simulink library "snn_champions_lib"  (R2026a)
settings: Solver=VariableStepAuto
(part 1 of 24)
settings Model: Creator=user poco smart  LastModifiedBy=user poco smart

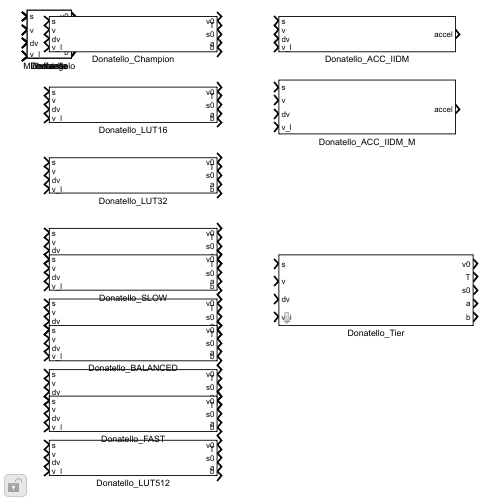
[thumbnail: Simulink's stored preview of the top-level diagram]
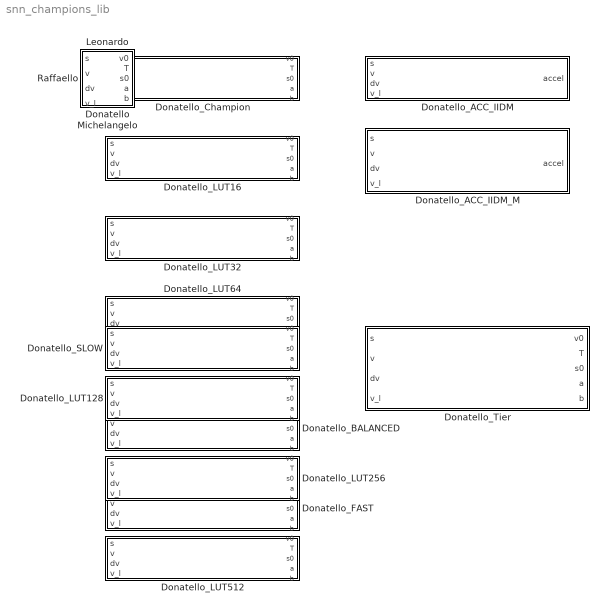
== system snn_champions_lib ==
  Donatello : Subsystem
  Donatello_ACC_IIDM : Subsystem  Description=|
      | Donatello_ACC_IIDM - campione Donatello (LUT-64) + modello ACC-IIDM open-loop.
      | 
      | HDL-READY dal 2026-07-16 (SP3): HDL Coder genera il VHDL dal solo .slx, con DualPortRAM (cioe'
      |    l'architettura time-mux del deployato). Fino a quella data l'IIDM girava in double e HDL
      |    Coder rifiutava il blocco con 14 errori; ora l'IIDM e' fixed-point (acc_types, Q10.8).
      |    Non servirono LUT: sqrt/tanh/x^4 sono NATIVI in HDL Coder e la divisione passa con
      |    RoundingMethod 'Zero'. Cancello: run_block_hdl_gate.
      | 
      | ⚠️ HDL-READY NON VUOL DIRE DEPLOYATO: il bitstream PYNQ-Z1 resta la sola SNN. Questo blocco da'
      |    il costo in silicio del controllore COMPLETO (rete + legge di controllo), che e' cio' che si
      |    confronta con un MPC. Dettagli: document/SP3_ACC_IIDM_HDL.md.
      | 
      | FUNZIONE
      |   Catena completa stato -> azione: la SNN stima i 5 parametri IDM, il modello ACC-IIDM li usa
      |   per calcolare l'accelerazione. Serve a testare la rete dentro un modello di car-following.
      | 
      | INGRESSI (fisici, fixed con >=20 bit frazionari - interporre un Data Type Conversion)
      |   s [m] · v [m/s] · dv [m/s] (= v - v_l) · v_l [m/s]
      | USCITA
      |   accel [m/s^2]
      | 
      | LOOP APERTO
      |   Il blocco NON integra v ne' s: li riceve. Il loop lo chiude il sistema che testa (la velocita'
      |   effettiva puo' essere alterata a valle). L'unico stato interno e' il filtro OU che stima a_l.
      | 
      | SEMANTICA E RATE
      |   1 cambio d'ingresso = 1 control-step = DT 0.1 s. Ogni ingresso va tenuto per almeno ~341
      |   campioni (la SNN e' time-multiplexata: 1 neurone/clock). L'IIDM gira una volta per
      |   control-step, quando i parametri si rinfrescano.
      | 
      | RIFERIMENTI
      |   docs/superpowers/specs/2026-07-14-sp2-donatello-acc-iidm-design.md · document/SP2_ACC_IIDM.md
      |   Rigenerazione: build_hdl_variants.m (NON modificare la chart a mano)
  Donatello_ACC_IIDM_M : Subsystem  Description=|
      | Donatello_ACC_IIDM_M - Donatello (LUT-64) + ACC-IIDM con le 5 divisioni SEQUENZIATE.
      | 
      | COS'E' (SP4-M-FSM #2a)
      |   Variante di Donatello_ACC_IIDM: le 5 divisioni a divisore variabile dell'IIDM non sono piu' 5
      |   divisori combinatori INCATENATI (1077 livelli logici, Fmax 2,0 MHz), ma UNA sola divide()
      |   riusata da una macchina a stati -- una divisione per ciclo. Scopo: TAGLIARE L'AREA tenendo
      |   dmax=0. Il path critico resta una divisione combinatoria: questo blocco NON punta agli 11,65 MHz
      |   (per quelli servirebbe un divisore sequenziale, studio #2b: SP4_ACC_IIDM_FAST.md).
      | 
      | BIT-IDENTICO A Donatello_ACC_IIDM (SP3)
      |   La matematica e' la stessa, solo distribuita nel tempo: nessuna approssimazione. Garantito da
      |   tre cancelli sul dataset intero:
      |     G1  il blocco Divide (ShiftAdd, RndMeth Zero, Q10.8) e' bit-identico a divide() di SP3
      |         -> dmax=0 su 300.000 coppie (num,den) reali; sensibile (RndMeth Nearest -> 1 LSB).
      |     G2  le funzioni-fase (iidm_prep/nd/use/final) == acc_iidm_open -> dmax=0 su 60.000/60.000
      |         control-step; sensibile (q2 al posto di q3 -> 1990/2000 divergenti).
      |     G3  questo blocco == il model acc_iidm_fsm (run_block_acciidm_m_test).
      | 
      | INGRESSI (fisici, fixed con >=20 bit frazionari - interporre un Data Type Conversion)
      |   s [m] · v [m/s] · dv [m/s] (= v - v_l) · v_l [m/s]
      | USCITA
      |   accel [m/s^2]
      | 
      | ⚠️ VINCOLO DI RATE (DIVERSO da Donatello_ACC_IIDM)
      |   Una inferenza costa la SNN time-mux (~341 clock) PIU' 5 cicli, uno per divisione. Ogni ingresso
      |   va quindi tenuto per PIU' campioni che nel blocco SP3 (~341): il valore esatto lo MISURA
      |   run_block_acciidm_m_test (non e' assunto). Sull'FPGA e' irrilevante: un control-step da 0,1 s
      |   dura 800.000 clock a 8 MHz.
      | 
      | SEMANTICA
      |   1 cambio d'ingresso = 1 inferenza (edge-triggered, niente start/done esposti: uno start
      |   scollegato sarebbe un fallimento SILENZIOSO -- HDL_PHASE §3.1.2). Le uscite mantengono l'ultimo
      |   valore fino all'inferenza successiva.
      | 
      | RIFERIMENTI
      |   docs/superpowers/specs/2026-07-16-acc-iidm-fsm-design.md · document/SP4_ACC_IIDM_FAST.md
      |   Rigenerazione: build_hdl_variants.m (NON modificare la chart a mano)
  Donatello_BALANCED : Subsystem  Description=|
      | Donatello_BALANCED - SNN car-following (champion Donatello), architettura SPLITPIPE (SNN+decode come due
      | entita' di sintesi, con registro sugli operandi del normalize). Tier dello Studio Trade-off (Blocco A).
      | 
      | CONFIGURAZIONE: R5 (SNN 5 stadi) + decode p3  -> tier COMPROMESSO (~58 MHz io-timed)
      | Decode della sigmoide via LUT a 64 punti. I tre tier danno gli STESSI 5 parametri (bit-exact fra loro),
      | differiscono per latenza (342/364/406 clock) e profilo di risorse/Fmax.
      | 
      | INGRESSI (fisici, fixed >=20 bit frazionari): s [m], v [m/s], dv [m/s] (sat +-20), v_l [m/s].
      | USCITE (parametri IDM): v0, T, s0, a, b.  1 campione = 1 inferenza (edge-triggered), niente start/done.
      | 
      | SELF-CONTAINED: nessun .m esterno; HDL Coder genera il VHDL dal solo blocco (time-mux, DualPortRAM).
      | VERIFICHE: run_block_hdl_gate (self-contained) · run_block_traj_test (dmax=0).
      | Rigenerazione: build_tier_blocks.m (NON modificare la chart a mano).
  Donatello_Champion : Subsystem  Description=|
      | Donatello_Champion - SNN car-following (champion Donatello), architettura B2 time-multiplexata.
      | 
      | FUNZIONE
      |   Stima i 5 parametri IDM del veicolo osservato a partire dallo stato di car-following.
      | 
      | INGRESSI (grandezze fisiche)
      |   s    [m]    spaziatura dal veicolo che precede
      |   v    [m/s]  velocita' del veicolo
      |   dv   [m/s]  velocita' relativa (v - v_l); saturata internamente a +-20
      |   v_l  [m/s]  velocita' del veicolo che precede
      | 
      | USCITE (parametri IDM stimati)
      |   v0 [m/s]  ·  T [s]  ·  s0 [m]  ·  a [m/s^2]  ·  b [m/s^2]
      | 
      | TIPI DI DATO (vincolo)
      |   Gli ingressi devono essere fixed-point con ALMENO 20 bit frazionari, ad esempio
      |   fixdt(1,32,20). Il tipo double NON e' ammesso: non e' sintetizzabile e il blocco non
      |   compila. Per sorgenti in double (es. le traiettorie di test_dataset.mat) interporre un
      |   blocco "Data Type Conversion". Con meno di 20 bit frazionari il blocco funziona ma non
      |   e' bit-exact rispetto al riferimento software (la normalizzazione devia di 1 LSB circa
      |   1 volta ogni 25 campioni, il che fa cambiare uno spike).
      | 
      | SEMANTICA: 1 campione = 1 inferenza
      |   Una inferenza viene avviata a ogni cambio degli ingressi (edge-triggered). Il blocco non
      |   espone start/done. Le uscite mantengono l'ultimo valore calcolato fino all'inferenza
      |   successiva.
      | 
      | VINCOLO DI RATE
      |   L'architettura time-multiplexata elabora un neurone per clock: una inferenza richiede
      |   circa 341 campioni. Ogni ingresso va quindi mantenuto per almeno 341 passi di simulazione.
      |   Il valore esatto e' irrilevante: qualunque durata >= 341 e' corretta. Sull'FPGA il vincolo
      |   e' soddisfatto con ampio margine (un control-step da 0.1 s dura 800.000 clock e l'inferenza
      |   ne usa 341, pari allo 0,04%).
      | 
      | LIMITE NOTO
      |   Se due campioni consecutivi hanno tutti e quattro gli ingressi bit-identici, il cambio non
      |   viene rilevato e una inferenza viene saltata.
      | 
      | IMPLEMENTAZIONE
      |   IL CAMPIONE: e' esattamente cio' che va sull'FPGA (stesso decode del top deployato snn_top_b2). Decode della sigmoide via LUT a 64 punti. Perche' 64: lo studio DECODE_LUT_SWEEP.md ha misurato che l'accuratezza e' piatta (~84%) su N=16..512, e che 64 e' la LUT piu' piccola il cui errore d'approssimazione su v0 (0.0114) resta SOTTO l'errore di quantizzazione fixed gia' accettato (0.028) -> il decode non diventa la fonte d'errore dominante. Rispetto ai 256 punti usati fino al 2026-07-14: accuratezza identica (83.98 vs 83.97) e -288 LUT sul top (4630 -> 4342). Nota: funzionalmente IDENTICO al blocco Donatello_LUT64 (qui il nome dice cosa si deploya, li' che e' una variante di studio).
      |   Il forward e' il B2 time-multiplexato, identico all'architettura del bitstream PYNQ-Z1.
      |   Il blocco e' SELF-CONTAINED: non richiede alcun file .m esterno. HDL Coder genera il VHDL
      |   direttamente dal blocco (architettura time-mux, con DualPortRAM).
      | 
      | VERIFICHE
      |   run_block_hdl_gate   - copia il solo .slx in una cartella isolata, rimuove matlab/ dal path
      |                          e lancia makehdl: dimostra che il VHDL si genera su un altro PC.
      |   run_block_traj_test  - pilota il blocco con le traiettorie di test_dataset.mat e verifica
      |                          che i parametri coincidano con il riferimento (dmax = 0).
      | 
      | RIFERIMENTI
      |   document/HDL_PHASE.md         §3.1 contratto d'interfaccia, §3.1.4 edge-trigger e rate
      |   document/DECODE_LUT_SWEEP.md  §6 blocchi e verifiche
      |   Rigenerazione: build_hdl_variants.m (NON modificare la chart a mano)
  Donatello_FAST : Subsystem  Description=|
      | Donatello_FAST - SNN car-following (champion Donatello), architettura SPLITPIPE (SNN+decode come due
      | entita' di sintesi, con registro sugli operandi del normalize). Tier dello Studio Trade-off (Blocco A).
      | 
      | CONFIGURAZIONE: R9 (SNN 9 stadi) + decode p5      -> tier MARGINE MASSIMO (~74 MHz io-timed)
      | Decode della sigmoide via LUT a 64 punti. I tre tier danno gli STESSI 5 parametri (bit-exact fra loro),
      | differiscono per latenza (342/364/406 clock) e profilo di risorse/Fmax.
      | 
      | INGRESSI (fisici, fixed >=20 bit frazionari): s [m], v [m/s], dv [m/s] (sat +-20), v_l [m/s].
      | USCITE (parametri IDM): v0, T, s0, a, b.  1 campione = 1 inferenza (edge-triggered), niente start/done.
      | 
      | SELF-CONTAINED: nessun .m esterno; HDL Coder genera il VHDL dal solo blocco (time-mux, DualPortRAM).
      | VERIFICHE: run_block_hdl_gate (self-contained) · run_block_traj_test (dmax=0).
      | Rigenerazione: build_tier_blocks.m (NON modificare la chart a mano).
  Donatello_LUT128 : Subsystem  Description=|
      | Donatello_LUT128 - SNN car-following (champion Donatello), architettura B2 time-multiplexata.
      | 
      | FUNZIONE
      |   Stima i 5 parametri IDM del veicolo osservato a partire dallo stato di car-following.
      | 
      | INGRESSI (grandezze fisiche)
      |   s    [m]    spaziatura dal veicolo che precede
      |   v    [m/s]  velocita' del veicolo
      |   dv   [m/s]  velocita' relativa (v - v_l); saturata internamente a +-20
      |   v_l  [m/s]  velocita' del veicolo che precede
      | 
      | USCITE (parametri IDM stimati)
      |   v0 [m/s]  ·  T [s]  ·  s0 [m]  ·  a [m/s^2]  ·  b [m/s^2]
      | 
      | TIPI DI DATO (vincolo)
      |   Gli ingressi devono essere fixed-point con ALMENO 20 bit frazionari, ad esempio
      |   fixdt(1,32,20). Il tipo double NON e' ammesso: non e' sintetizzabile e il blocco non
      |   compila. Per sorgenti in double (es. le traiettorie di test_dataset.mat) interporre un
      |   blocco "Data Type Conversion". Con meno di 20 bit frazionari il blocco funziona ma non
      |   e' bit-exact rispetto al riferimento software (la normalizzazione devia di 1 LSB circa
      |   1 volta ogni 25 campioni, il che fa cambiare uno spike).
      | 
      | SEMANTICA: 1 campione = 1 inferenza
      |   Una inferenza viene avviata a ogni cambio degli ingressi (edge-triggered). Il blocco non
      |   espone start/done. Le uscite mantengono l'ultimo valore calcolato fino all'inferenza
      |   successiva.
      | 
      | VINCOLO DI RATE
      |   L'architettura time-multiplexata elabora un neurone per clock: una inferenza richiede
      |   circa 341 campioni. Ogni ingresso va quindi mantenuto per almeno 341 passi di simulazione.
      |   Il valore esatto e' irrilevante: qualunque durata >= 341 e' corretta. Sull'FPGA il vincolo
      |   e' soddisfatto con ampio margine (un control-step da 0.1 s dura 800.000 clock e l'inferenza
      |   ne usa 341, pari allo 0,04%).
      | 
      | LIMITE NOTO
      |   Se due campioni consecutivi hanno tutti e quattro gli ingressi bit-identici, il cambio non
      |   viene rilevato e una inferenza viene saltata.
      | 
      | IMPLEMENTAZIONE
      |   Decode della sigmoide via LUT a 128 punti (snn_decode_lut). Variante per lo studio del compromesso dimensione-LUT / accuratezza / risorse: l'accuratezza e' piatta (~84%) su N=16..512 mentre le LUT di sintesi crescono da 520 a 1732 (vedi document/DECODE_LUT_SWEEP.md). Il forward e' identico in tutte le varianti.
      |   Il forward e' il B2 time-multiplexato, identico all'architettura del bitstream PYNQ-Z1.
      |   Il blocco e' SELF-CONTAINED: non richiede alcun file .m esterno. HDL Coder genera il VHDL
      |   direttamente dal blocco (architettura time-mux, con DualPortRAM).
      | 
      | VERIFICHE
      |   run_block_hdl_gate   - copia il solo .slx in una cartella isolata, rimuove matlab/ dal path
      |                          e lancia makehdl: dimostra che il VHDL si genera su un altro PC.
      |   run_block_traj_test  - pilota il blocco con le traiettorie di test_dataset.mat e verifica
      |                          che i parametri coincidano con il riferimento (dmax = 0).
      | 
      | RIFERIMENTI
      |   document/HDL_PHASE.md         §3.1 contratto d'interfaccia, §3.1.4 edge-trigger e rate
      |   document/DECODE_LUT_SWEEP.md  §6 blocchi e verifiche
      |   Rigenerazione: build_hdl_variants.m (NON modificare la chart a mano)
  Donatello_LUT16 : Subsystem  Description=|
      | Donatello_LUT16 - SNN car-following (champion Donatello), architettura B2 time-multiplexata.
      | 
      | FUNZIONE
      |   Stima i 5 parametri IDM del veicolo osservato a partire dallo stato di car-following.
      | 
      | INGRESSI (grandezze fisiche)
      |   s    [m]    spaziatura dal veicolo che precede
      |   v    [m/s]  velocita' del veicolo
      |   dv   [m/s]  velocita' relativa (v - v_l); saturata internamente a +-20
      |   v_l  [m/s]  velocita' del veicolo che precede
      | 
      | USCITE (parametri IDM stimati)
      |   v0 [m/s]  ·  T [s]  ·  s0 [m]  ·  a [m/s^2]  ·  b [m/s^2]
      | 
      | TIPI DI DATO (vincolo)
      |   Gli ingressi devono essere fixed-point con ALMENO 20 bit frazionari, ad esempio
      |   fixdt(1,32,20). Il tipo double NON e' ammesso: non e' sintetizzabile e il blocco non
      |   compila. Per sorgenti in double (es. le traiettorie di test_dataset.mat) interporre un
      |   blocco "Data Type Conversion". Con meno di 20 bit frazionari il blocco funziona ma non
      |   e' bit-exact rispetto al riferimento software (la normalizzazione devia di 1 LSB circa
      |   1 volta ogni 25 campioni, il che fa cambiare uno spike).
      | 
      | SEMANTICA: 1 campione = 1 inferenza
      |   Una inferenza viene avviata a ogni cambio degli ingressi (edge-triggered). Il blocco non
      |   espone start/done. Le uscite mantengono l'ultimo valore calcolato fino all'inferenza
      |   successiva.
      | 
      | VINCOLO DI RATE
      |   L'architettura time-multiplexata elabora un neurone per clock: una inferenza richiede
      |   circa 341 campioni. Ogni ingresso va quindi mantenuto per almeno 341 passi di simulazione.
      |   Il valore esatto e' irrilevante: qualunque durata >= 341 e' corretta. Sull'FPGA il vincolo
      |   e' soddisfatto con ampio margine (un control-step da 0.1 s dura 800.000 clock e l'inferenza
      |   ne usa 341, pari allo 0,04%).
      | 
      | LIMITE NOTO
      |   Se due campioni consecutivi hanno tutti e quattro gli ingressi bit-identici, il cambio non
      |   viene rilevato e una inferenza viene saltata.
      | 
      | IMPLEMENTAZIONE
      |   Decode della sigmoide via LUT a 16 punti (snn_decode_lut). Variante per lo studio del compromesso dimensione-LUT / accuratezza / risorse: l'accuratezza e' piatta (~84%) su N=16..512 mentre le LUT di sintesi crescono da 520 a 1732 (vedi document/DECODE_LUT_SWEEP.md). Il forward e' identico in tutte le varianti.
      |   Il forward e' il B2 time-multiplexato, identico all'architettura del bitstream PYNQ-Z1.
      |   Il blocco e' SELF-CONTAINED: non richiede alcun file .m esterno. HDL Coder genera il VHDL
      |   direttamente dal blocco (architettura time-mux, con DualPortRAM).
      | 
      | VERIFICHE
      |   run_block_hdl_gate   - copia il solo .slx in una cartella isolata, rimuove matlab/ dal path
      |                          e lancia makehdl: dimostra che il VHDL si genera su un altro PC.
      |   run_block_traj_test  - pilota il blocco con le traiettorie di test_dataset.mat e verifica
      |                          che i parametri coincidano con il riferimento (dmax = 0).
      | 
      | RIFERIMENTI
      |   document/HDL_PHASE.md         §3.1 contratto d'interfaccia, §3.1.4 edge-trigger e rate
      |   document/DECODE_LUT_SWEEP.md  §6 blocchi e verifiche
      |   Rigenerazione: build_hdl_variants.m (NON modificare la chart a mano)
  Donatello_LUT256 : Subsystem  Description=|
      | Donatello_LUT256 - SNN car-following (champion Donatello), architettura B2 time-multiplexata.
      | 
      | FUNZIONE
      |   Stima i 5 parametri IDM del veicolo osservato a partire dallo stato di car-following.
      | 
      | INGRESSI (grandezze fisiche)
      |   s    [m]    spaziatura dal veicolo che precede
      |   v    [m/s]  velocita' del veicolo
      |   dv   [m/s]  velocita' relativa (v - v_l); saturata internamente a +-20
      |   v_l  [m/s]  velocita' del veicolo che precede
      | 
      | USCITE (parametri IDM stimati)
      |   v0 [m/s]  ·  T [s]  ·  s0 [m]  ·  a [m/s^2]  ·  b [m/s^2]
      | 
      | TIPI DI DATO (vincolo)
      |   Gli ingressi devono essere fixed-point con ALMENO 20 bit frazionari, ad esempio
      |   fixdt(1,32,20). Il tipo double NON e' ammesso: non e' sintetizzabile e il blocco non
      |   compila. Per sorgenti in double (es. le traiettorie di test_dataset.mat) interporre un
      |   blocco "Data Type Conversion". Con meno di 20 bit frazionari il blocco funziona ma non
      |   e' bit-exact rispetto al riferimento software (la normalizzazione devia di 1 LSB circa
      |   1 volta ogni 25 campioni, il che fa cambiare uno spike).
      | 
      | SEMANTICA: 1 campione = 1 inferenza
      |   Una inferenza viene avviata a ogni cambio degli ingressi (edge-triggered). Il blocco non
      |   espone start/done. Le uscite mantengono l'ultimo valore calcolato fino all'inferenza
      |   successiva.
      | 
      | VINCOLO DI RATE
      |   L'architettura time-multiplexata elabora un neurone per clock: una inferenza richiede
      |   circa 341 campioni. Ogni ingresso va quindi mantenuto per almeno 341 passi di simulazione.
      |   Il valore esatto e' irrilevante: qualunque durata >= 341 e' corretta. Sull'FPGA il vincolo
      |   e' soddisfatto con ampio margine (un control-step da 0.1 s dura 800.000 clock e l'inferenza
      |   ne usa 341, pari allo 0,04%).
      | 
      | LIMITE NOTO
      |   Se due campioni consecutivi hanno tutti e quattro gli ingressi bit-identici, il cambio non
      |   viene rilevato e una inferenza viene saltata.
      | 
      | IMPLEMENTAZIONE
      |   Decode della sigmoide via LUT a 256 punti (snn_decode_lut). Variante per lo studio del compromesso dimensione-LUT / accuratezza / risorse: l'accuratezza e' piatta (~84%) su N=16..512 mentre le LUT di sintesi crescono da 520 a 1732 (vedi document/DECODE_LUT_SWEEP.md). Il forward e' identico in tutte le varianti.
      |   Il forward e' il B2 time-multiplexato, identico all'architettura del bitstream PYNQ-Z1.
      |   Il blocco e' SELF-CONTAINED: non richiede alcun file .m esterno. HDL Coder genera il VHDL
      |   direttamente dal blocco (architettura time-mux, con DualPortRAM).
      | 
      | VERIFICHE
      |   run_block_hdl_gate   - copia il solo .slx in una cartella isolata, rimuove matlab/ dal path
      |                          e lancia makehdl: dimostra che il VHDL si genera su un altro PC.
      |   run_block_traj_test  - pilota il blocco con le traiettorie di test_dataset.mat e verifica
      |                          che i parametri coincidano con il riferimento (dmax = 0).
      | 
      | RIFERIMENTI
      |   document/HDL_PHASE.md         §3.1 contratto d'interfaccia, §3.1.4 edge-trigger e rate
      |   document/DECODE_LUT_SWEEP.md  §6 blocchi e verifiche
      |   Rigenerazione: build_hdl_variants.m (NON modificare la chart a mano)
  Donatello_LUT32 : Subsystem  Description=|
      | Donatello_LUT32 - SNN car-following (champion Donatello), architettura B2 time-multiplexata.
      | 
      | FUNZIONE
      |   Stima i 5 parametri IDM del veicolo osservato a partire dallo stato di car-following.
      | 
      | INGRESSI (grandezze fisiche)
      |   s    [m]    spaziatura dal veicolo che precede
      |   v    [m/s]  velocita' del veicolo
      |   dv   [m/s]  velocita' relativa (v - v_l); saturata internamente a +-20
      |   v_l  [m/s]  velocita' del veicolo che precede
      | 
      | USCITE (parametri IDM stimati)
      |   v0 [m/s]  ·  T [s]  ·  s0 [m]  ·  a [m/s^2]  ·  b [m/s^2]
      | 
      | TIPI DI DATO (vincolo)
      |   Gli ingressi devono essere fixed-point con ALMENO 20 bit frazionari, ad esempio
      |   fixdt(1,32,20). Il tipo double NON e' ammesso: non e' sintetizzabile e il blocco non
      |   compila. Per sorgenti in double (es. le traiettorie di test_dataset.mat) interporre un
      |   blocco "Data Type Conversion". Con meno di 20 bit frazionari il blocco funziona ma non
      |   e' bit-exact rispetto al riferimento software (la normalizzazione devia di 1 LSB circa
      |   1 volta ogni 25 campioni, il che fa cambiare uno spike).
      | 
      | SEMANTICA: 1 campione = 1 inferenza
      |   Una inferenza viene avviata a ogni cambio degli ingressi (edge-triggered). Il blocco non
      |   espone start/done. Le uscite mantengono l'ultimo valore calcolato fino all'inferenza
      |   successiva.
      | 
      | VINCOLO DI RATE
      |   L'architettura time-multiplexata elabora un neurone per clock: una inferenza richiede
      |   circa 341 campioni. Ogni ingresso va quindi mantenuto per almeno 341 passi di simulazione.
      |   Il valore esatto e' irrilevante: qualunque durata >= 341 e' corretta. Sull'FPGA il vincolo
      |   e' soddisfatto con ampio margine (un control-step da 0.1 s dura 800.000 clock e l'inferenza
      |   ne usa 341, pari allo 0,04%).
      | 
      | LIMITE NOTO
      |   Se due campioni consecutivi hanno tutti e quattro gli ingressi bit-identici, il cambio non
      |   viene rilevato e una inferenza viene saltata.
      | 
      | IMPLEMENTAZIONE
      |   Decode della sigmoide via LUT a 32 punti (snn_decode_lut). Variante per lo studio del compromesso dimensione-LUT / accuratezza / risorse: l'accuratezza e' piatta (~84%) su N=16..512 mentre le LUT di sintesi crescono da 520 a 1732 (vedi document/DECODE_LUT_SWEEP.md). Il forward e' identico in tutte le varianti.
      |   Il forward e' il B2 time-multiplexato, identico all'architettura del bitstream PYNQ-Z1.
      |   Il blocco e' SELF-CONTAINED: non richiede alcun file .m esterno. HDL Coder genera il VHDL
      |   direttamente dal blocco (architettura time-mux, con DualPortRAM).
      | 
      | VERIFICHE
      |   run_block_hdl_gate   - copia il solo .slx in una cartella isolata, rimuove matlab/ dal path
      |                          e lancia makehdl: dimostra che il VHDL si genera su un altro PC.
      |   run_block_traj_test  - pilota il blocco con le traiettorie di test_dataset.mat e verifica
      |                          che i parametri coincidano con il riferimento (dmax = 0).
      | 
      | RIFERIMENTI
      |   document/HDL_PHASE.md         §3.1 contratto d'interfaccia, §3.1.4 edge-trigger e rate
      |   document/DECODE_LUT_SWEEP.md  §6 blocchi e verifiche
      |   Rigenerazione: build_hdl_variants.m (NON modificare la chart a mano)
  Donatello_LUT512 : Subsystem  Description=|
      | Donatello_LUT512 - SNN car-following (champion Donatello), architettura B2 time-multiplexata.
      | 
      | FUNZIONE
      |   Stima i 5 parametri IDM del veicolo osservato a partire dallo stato di car-following.
      | 
      | INGRESSI (grandezze fisiche)
      |   s    [m]    spaziatura dal veicolo che precede
      |   v    [m/s]  velocita' del veicolo
      |   dv   [m/s]  velocita' relativa (v - v_l); saturata internamente a +-20
      |   v_l  [m/s]  velocita' del veicolo che precede
      | 
      | USCITE (parametri IDM stimati)
      |   v0 [m/s]  ·  T [s]  ·  s0 [m]  ·  a [m/s^2]  ·  b [m/s^2]
      | 
      | TIPI DI DATO (vincolo)
      |   Gli ingressi devono essere fixed-point con ALMENO 20 bit frazionari, ad esempio
      |   fixdt(1,32,20). Il tipo double NON e' ammesso: non e' sintetizzabile e il blocco non
      |   compila. Per sorgenti in double (es. le traiettorie di test_dataset.mat) interporre un
      |   blocco "Data Type Conversion". Con meno di 20 bit frazionari il blocco funziona ma non
      |   e' bit-exact rispetto al riferimento software (la normalizzazione devia di 1 LSB circa
      |   1 volta ogni 25 campioni, il che fa cambiare uno spike).
      | 
      | SEMANTICA: 1 campione = 1 inferenza
      |   Una inferenza viene avviata a ogni cambio degli ingressi (edge-triggered). Il blocco non
      |   espone start/done. Le uscite mantengono l'ultimo valore calcolato fino all'inferenza
      |   successiva.
      | 
      | VINCOLO DI RATE
      |   L'architettura time-multiplexata elabora un neurone per clock: una inferenza richiede
      |   circa 341 campioni. Ogni ingresso va quindi mantenuto per almeno 341 passi di simulazione.
      |   Il valore esatto e' irrilevante: qualunque durata >= 341 e' corretta. Sull'FPGA il vincolo
      |   e' soddisfatto con ampio margine (un control-step da 0.1 s dura 800.000 clock e l'inferenza
      |   ne usa 341, pari allo 0,04%).
      | 
      | LIMITE NOTO
      |   Se due campioni consecutivi hanno tutti e quattro gli ingressi bit-identici, il cambio non
      |   viene rilevato e una inferenza viene saltata.
      | 
      | IMPLEMENTAZIONE
      |   Decode della sigmoide via LUT a 512 punti (snn_decode_lut). Variante per lo studio del compromesso dimensione-LUT / accuratezza / risorse: l'accuratezza e' piatta (~84%) su N=16..512 mentre le LUT di sintesi crescono da 520 a 1732 (vedi document/DECODE_LUT_SWEEP.md). Il forward e' identico in tutte le varianti.
      |   Il forward e' il B2 time-multiplexato, identico all'architettura del bitstream PYNQ-Z1.
      |   Il blocco e' SELF-CONTAINED: non richiede alcun file .m esterno. HDL Coder genera il VHDL
      |   direttamente dal blocco (architettura time-mux, con DualPortRAM).
      | 
      | VERIFICHE
      |   run_block_hdl_gate   - copia il solo .slx in una cartella isolata, rimuove matlab/ dal path
      |                          e lancia makehdl: dimostra che il VHDL si genera su un altro PC.
      |   run_block_traj_test  - pilota il blocco con le traiettorie di test_dataset.mat e verifica
      |                          che i parametri coincidano con il riferimento (dmax = 0).
      | 
      | RIFERIMENTI
      |   document/HDL_PHASE.md         §3.1 contratto d'interfaccia, §3.1.4 edge-trigger e rate
      |   document/DECODE_LUT_SWEEP.md  §6 blocchi e verifiche
      |   Rigenerazione: build_hdl_variants.m (NON modificare la chart a mano)
  Donatello_LUT64 : Subsystem  Description=|
      | Donatello_LUT64 - SNN car-following (champion Donatello), architettura B2 time-multiplexata.
      | 
      | FUNZIONE
      |   Stima i 5 parametri IDM del veicolo osservato a partire dallo stato di car-following.
      | 
      | INGRESSI (grandezze fisiche)
      |   s    [m]    spaziatura dal veicolo che precede
      |   v    [m/s]  velocita' del veicolo
      |   dv   [m/s]  velocita' relativa (v - v_l); saturata internamente a +-20
      |   v_l  [m/s]  velocita' del veicolo che precede
      | 
      | USCITE (parametri IDM stimati)
      |   v0 [m/s]  ·  T [s]  ·  s0 [m]  ·  a [m/s^2]  ·  b [m/s^2]
      | 
      | TIPI DI DATO (vincolo)
      |   Gli ingressi devono essere fixed-point con ALMENO 20 bit frazionari, ad esempio
      |   fixdt(1,32,20). Il tipo double NON e' ammesso: non e' sintetizzabile e il blocco non
      |   compila. Per sorgenti in double (es. le traiettorie di test_dataset.mat) interporre un
      |   blocco "Data Type Conversion". Con meno di 20 bit frazionari il blocco funziona ma non
      |   e' bit-exact rispetto al riferimento software (la normalizzazione devia di 1 LSB circa
      |   1 volta ogni 25 campioni, il che fa cambiare uno spike).
      | 
      | SEMANTICA: 1 campione = 1 inferenza
      |   Una inferenza viene avviata a ogni cambio degli ingressi (edge-triggered). Il blocco non
      |   espone start/done. Le uscite mantengono l'ultimo valore calcolato fino all'inferenza
      |   successiva.
      | 
      | VINCOLO DI RATE
      |   L'architettura time-multiplexata elabora un neurone per clock: una inferenza richiede
      |   circa 341 campioni. Ogni ingresso va quindi mantenuto per almeno 341 passi di simulazione.
      |   Il valore esatto e' irrilevante: qualunque durata >= 341 e' corretta. Sull'FPGA il vincolo
      |   e' soddisfatto con ampio margine (un control-step da 0.1 s dura 800.000 clock e l'inferenza
      |   ne usa 341, pari allo 0,04%).
      | 
      | LIMITE NOTO
      |   Se due campioni consecutivi hanno tutti e quattro gli ingressi bit-identici, il cambio non
      |   viene rilevato e una inferenza viene saltata.
      | 
      | IMPLEMENTAZIONE
      |   Decode della sigmoide via LUT a 64 punti (snn_decode_lut). Variante per lo studio del compromesso dimensione-LUT / accuratezza / risorse: l'accuratezza e' piatta (~84%) su N=16..512 mentre le LUT di sintesi crescono da 520 a 1732 (vedi document/DECODE_LUT_SWEEP.md). Il forward e' identico in tutte le varianti.
      |   Il forward e' il B2 time-multiplexato, identico all'architettura del bitstream PYNQ-Z1.
      |   Il blocco e' SELF-CONTAINED: non richiede alcun file .m esterno. HDL Coder genera il VHDL
      |   direttamente dal blocco (architettura time-mux, con DualPortRAM).
      | 
      | VERIFICHE
      |   run_block_hdl_gate   - copia il solo .slx in una cartella isolata, rimuove matlab/ dal path
      |                          e lancia makehdl: dimostra che il VHDL si genera su un altro PC.
      |   run_block_traj_test  - pilota il blocco con le traiettorie di test_dataset.mat e verifica
      |                          che i parametri coincidano con il riferimento (dmax = 0).
      | 
      | RIFERIMENTI
      |   document/HDL_PHASE.md         §3.1 contratto d'interfaccia, §3.1.4 edge-trigger e rate
      |   document/DECODE_LUT_SWEEP.md  §6 blocchi e verifiche
      |   Rigenerazione: build_hdl_variants.m (NON modificare la chart a mano)
  Donatello_SLOW : Subsystem  Description=|
      | Donatello_SLOW - SNN car-following (champion Donatello), architettura SPLITPIPE (SNN+decode come due
      | entita' di sintesi, con registro sugli operandi del normalize). Tier dello Studio Trade-off (Blocco A).
      | 
      | CONFIGURAZIONE: R2 (SNN 2 stadi) + decode fused  -> tier AREA MINIMA (~30 MHz io-timed)
      | Decode della sigmoide via LUT a 64 punti. I tre tier danno gli STESSI 5 parametri (bit-exact fra loro),
      | differiscono per latenza (342/364/406 clock) e profilo di risorse/Fmax.
      | 
      | INGRESSI (fisici, fixed >=20 bit frazionari): s [m], v [m/s], dv [m/s] (sat +-20), v_l [m/s].
      | USCITE (parametri IDM): v0, T, s0, a, b.  1 campione = 1 inferenza (edge-triggered), niente start/done.
      | 
      | SELF-CONTAINED: nessun .m esterno; HDL Coder genera il VHDL dal solo blocco (time-mux, DualPortRAM).
      | VERIFICHE: run_block_hdl_gate (self-contained) · run_block_traj_test (dmax=0).
      | Rigenerazione: build_tier_blocks.m (NON modificare la chart a mano).
  Donatello_Tier : Subsystem  mask{TIER=BALANCED, NFRAC=13, ADV=off, nV=13, nfat=13, nacc=13, naccw=13, nraw=13, nw=13}
      mask prompts: TIER "Tier (trade-off area/margine)"; NFRAC "nfrac Base (13 pieno / 8 / 5 / 2)"; ADV "Modalita' Avanzata (nfrac per-campo)"; nV "nfrac V (membrana)"; nfat "nfrac fatigue (soglia)"; nacc "nfrac acc (ingresso)"; naccw "nfrac accw (wide)"; nraw "nfrac raw (readout)"; nw "nfrac w (pesi po2)"
      mask help:
      | Donatello_Tier - SNN car-following (champion Donatello) CONFIGURABILE.
      | Un blocco, due modi. BASE: menu TIER (SLOW/BALANCED/FAST) + NFRAC (13/8/5/2). AVANZATO: checkbox ADV +
      | 6 slider nfrac per-campo. La selezione attiva la variante (Variant Subsystem, update diagram): HDL Coder
      | genera SOLO la variante scelta, coi tipi fixed-point gia' cotti.
      |
      | TIER: SLOW = R2/fused (area minima) · BALANCED = R5/p3 · FAST = R9/p5 (margine massimo).
      |
      | NFRAC (Base): bit frazionari UNICI del core SNN. 13=piena precisione (bit-exact) · 8 · 5 · 2 (safety-only).
      |
      | MODALITA' AVANZATA (ADV): 6 nfrac indipendenti [V fatigue acc accw raw w]. Gli slider MOSTRANO la config
      | attualmente COTTA nella variante ADV. Studio quantizzazione per-campo: acc/w scendibili a 4 bit
      | bit-exact (pesi po2, min 2^-4); V/fatigue/accw/raw servono pieni sotto il cancello 0.5 m. Config
      | area-ottimale = [13 13 4 13 13 4].
      | PER CAMBIARE la config ADV: esegui  build_tier_configurable([nV nfat nacc naccw nraw nw])  (ri-cuoce la
      | variante ADV a quei valori). Gli slider sono il valore da passare; la loro modifica nella mask NON ri-cuoce
      | da sola (un blocco linkato non si auto-rigenera: si passa dal builder).
      |
      | I/O fisico (fixed >=20 bit frazionari): s,v,dv,v_l -> v0,T,s0,a,b. Edge-triggered. Self-contained.
      | Richiede matlab/ sul path (callback tier_adv_cb). Rigenerazione: build_tier_configurable.m.
      mask TypeOptions TIER: SLOW | BALANCED | FAST
      mask TypeOptions NFRAC: 13 | 8 | 5 | 2
      mask Callback ADV: tier_adv_cb(gcb)
  Leonardo : Subsystem
  Michelangelo : Subsystem
  Raffaello : Subsystem

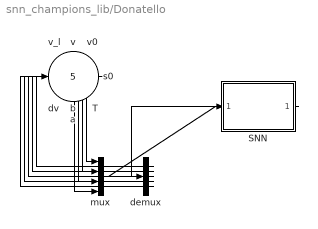
== system snn_champions_lib/Donatello ==
  s : Inport
  v : Inport  Port=2
  dv : Inport  Port=3
  v_l : Inport  Port=4
  SNN : MATLAB Function  TreatAsAtomicUnit=on
  demux : Demux  Outputs=5
  mux : Mux
  v0 : Outport
  T : Outport  Port=2
  s0 : Outport  Port=3
  a : Outport  Port=4
  b : Outport  Port=5
  wires:
  s/1 -> mux/1
  v/1 -> mux/2
  dv/1 -> mux/3
  v_l/1 -> mux/4
  mux/1 -> SNN/1(x_phys)
  SNN/1(params) -> demux/1
  demux/1 -> v0/1
  demux/2 -> T/1
  demux/3 -> s0/1
  demux/4 -> a/1
  demux/5 -> b/1

== system snn_champions_lib/Donatello_ACC_IIDM ==
  s : Inport
  v : Inport  Port=2
  dv : Inport  Port=3
  v_l : Inport  Port=4
  SNN_ACC : MATLAB Function  TreatAsAtomicUnit=on
  accel : Outport
  wires:
  s/1 -> SNN_ACC/1(s)
  v/1 -> SNN_ACC/2(v)
  dv/1 -> SNN_ACC/3(dv)
  v_l/1 -> SNN_ACC/4(v_l)
  SNN_ACC/1(accel) -> accel/1

== system snn_champions_lib/Donatello_ACC_IIDM_M ==
  s : Inport
  v : Inport  Port=2
  dv : Inport  Port=3
  v_l : Inport  Port=4
  IIDM_CTRL : MATLAB Function  TreatAsAtomicUnit=on
  accel : Outport
  wires:
  s/1 -> IIDM_CTRL/1(s)
  v/1 -> IIDM_CTRL/2(v)
  dv/1 -> IIDM_CTRL/3(dv)
  v_l/1 -> IIDM_CTRL/4(v_l)
  IIDM_CTRL/1(accel) -> accel/1

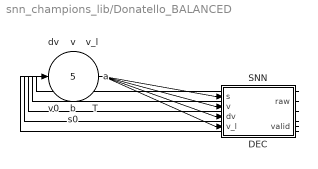
== system snn_champions_lib/Donatello_BALANCED ==
  s : Inport
  v : Inport  Port=2
  dv : Inport  Port=3
  v_l : Inport  Port=4
  DEC : MATLAB Function  TreatAsAtomicUnit=on
  SNN : MATLAB Function  TreatAsAtomicUnit=on
  v0 : Outport
  T : Outport  Port=2
  s0 : Outport  Port=3
  a : Outport  Port=4
  b : Outport  Port=5
  wires:
  s/1 -> SNN/1(s)
  v/1 -> SNN/2(v)
  dv/1 -> SNN/3(dv)
  v_l/1 -> SNN/4(v_l)
  SNN/1(raw) -> DEC/1(raw)
  SNN/2(valid) -> DEC/2(valid)
  DEC/1(v0) -> v0/1
  DEC/2(T) -> T/1
  DEC/3(s0) -> s0/1
  DEC/4(a) -> a/1
  DEC/5(b) -> b/1

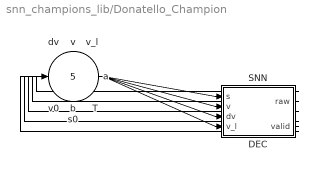
== system snn_champions_lib/Donatello_Champion ==
  s : Inport
  v : Inport  Port=2
  dv : Inport  Port=3
  v_l : Inport  Port=4
  DEC : MATLAB Function  TreatAsAtomicUnit=on
  SNN : MATLAB Function  TreatAsAtomicUnit=on
  v0 : Outport
  T : Outport  Port=2
  s0 : Outport  Port=3
  a : Outport  Port=4
  b : Outport  Port=5
  wires:
  s/1 -> SNN/1(s)
  v/1 -> SNN/2(v)
  dv/1 -> SNN/3(dv)
  v_l/1 -> SNN/4(v_l)
  SNN/1(raw) -> DEC/1(raw)
  SNN/2(valid) -> DEC/2(valid)
  DEC/1(v0) -> v0/1
  DEC/2(T) -> T/1
  DEC/3(s0) -> s0/1
  DEC/4(a) -> a/1
  DEC/5(b) -> b/1

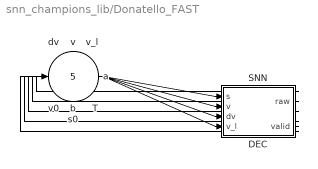
== system snn_champions_lib/Donatello_FAST ==
  s : Inport
  v : Inport  Port=2
  dv : Inport  Port=3
  v_l : Inport  Port=4
  DEC : MATLAB Function  TreatAsAtomicUnit=on
  SNN : MATLAB Function  TreatAsAtomicUnit=on
  v0 : Outport
  T : Outport  Port=2
  s0 : Outport  Port=3
  a : Outport  Port=4
  b : Outport  Port=5
  wires:
  s/1 -> SNN/1(s)
  v/1 -> SNN/2(v)
  dv/1 -> SNN/3(dv)
  v_l/1 -> SNN/4(v_l)
  SNN/1(raw) -> DEC/1(raw)
  SNN/2(valid) -> DEC/2(valid)
  DEC/1(v0) -> v0/1
  DEC/2(T) -> T/1
  DEC/3(s0) -> s0/1
  DEC/4(a) -> a/1
  DEC/5(b) -> b/1

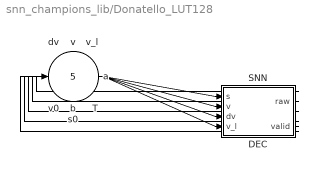
== system snn_champions_lib/Donatello_LUT128 ==
  s : Inport
  v : Inport  Port=2
  dv : Inport  Port=3
  v_l : Inport  Port=4
  DEC : MATLAB Function  TreatAsAtomicUnit=on
  SNN : MATLAB Function  TreatAsAtomicUnit=on
  v0 : Outport
  T : Outport  Port=2
  s0 : Outport  Port=3
  a : Outport  Port=4
  b : Outport  Port=5
  wires:
  s/1 -> SNN/1(s)
  v/1 -> SNN/2(v)
  dv/1 -> SNN/3(dv)
  v_l/1 -> SNN/4(v_l)
  SNN/1(raw) -> DEC/1(raw)
  SNN/2(valid) -> DEC/2(valid)
  DEC/1(v0) -> v0/1
  DEC/2(T) -> T/1
  DEC/3(s0) -> s0/1
  DEC/4(a) -> a/1
  DEC/5(b) -> b/1

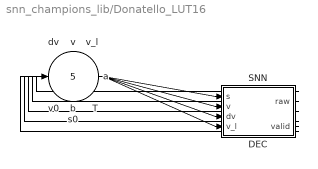
== system snn_champions_lib/Donatello_LUT16 ==
  s : Inport
  v : Inport  Port=2
  dv : Inport  Port=3
  v_l : Inport  Port=4
  DEC : MATLAB Function  TreatAsAtomicUnit=on
  SNN : MATLAB Function  TreatAsAtomicUnit=on
  v0 : Outport
  T : Outport  Port=2
  s0 : Outport  Port=3
  a : Outport  Port=4
  b : Outport  Port=5
  wires:
  s/1 -> SNN/1(s)
  v/1 -> SNN/2(v)
  dv/1 -> SNN/3(dv)
  v_l/1 -> SNN/4(v_l)
  SNN/1(raw) -> DEC/1(raw)
  SNN/2(valid) -> DEC/2(valid)
  DEC/1(v0) -> v0/1
  DEC/2(T) -> T/1
  DEC/3(s0) -> s0/1
  DEC/4(a) -> a/1
  DEC/5(b) -> b/1

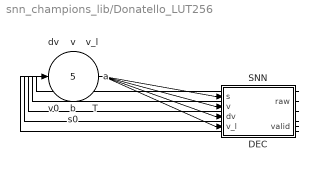
== system snn_champions_lib/Donatello_LUT256 ==
  s : Inport
  v : Inport  Port=2
  dv : Inport  Port=3
  v_l : Inport  Port=4
  DEC : MATLAB Function  TreatAsAtomicUnit=on
  SNN : MATLAB Function  TreatAsAtomicUnit=on
  v0 : Outport
  T : Outport  Port=2
  s0 : Outport  Port=3
  a : Outport  Port=4
  b : Outport  Port=5
  wires:
  s/1 -> SNN/1(s)
  v/1 -> SNN/2(v)
  dv/1 -> SNN/3(dv)
  v_l/1 -> SNN/4(v_l)
  SNN/1(raw) -> DEC/1(raw)
  SNN/2(valid) -> DEC/2(valid)
  DEC/1(v0) -> v0/1
  DEC/2(T) -> T/1
  DEC/3(s0) -> s0/1
  DEC/4(a) -> a/1
  DEC/5(b) -> b/1

== system snn_champions_lib/Donatello_LUT32 ==
  s : Inport
  v : Inport  Port=2
  dv : Inport  Port=3
  v_l : Inport  Port=4
  DEC : MATLAB Function  TreatAsAtomicUnit=on
  SNN : MATLAB Function  TreatAsAtomicUnit=on
  v0 : Outport
  T : Outport  Port=2
  s0 : Outport  Port=3
  a : Outport  Port=4
  b : Outport  Port=5
  wires:
  s/1 -> SNN/1(s)
  v/1 -> SNN/2(v)
  dv/1 -> SNN/3(dv)
  v_l/1 -> SNN/4(v_l)
  SNN/1(raw) -> DEC/1(raw)
  SNN/2(valid) -> DEC/2(valid)
  DEC/1(v0) -> v0/1
  DEC/2(T) -> T/1
  DEC/3(s0) -> s0/1
  DEC/4(a) -> a/1
  DEC/5(b) -> b/1

== system snn_champions_lib/Donatello_LUT512 ==
  s : Inport
  v : Inport  Port=2
  dv : Inport  Port=3
  v_l : Inport  Port=4
  DEC : MATLAB Function  TreatAsAtomicUnit=on
  SNN : MATLAB Function  TreatAsAtomicUnit=on
  v0 : Outport
  T : Outport  Port=2
  s0 : Outport  Port=3
  a : Outport  Port=4
  b : Outport  Port=5
  wires:
  s/1 -> SNN/1(s)
  v/1 -> SNN/2(v)
  dv/1 -> SNN/3(dv)
  v_l/1 -> SNN/4(v_l)
  SNN/1(raw) -> DEC/1(raw)
  SNN/2(valid) -> DEC/2(valid)
  DEC/1(v0) -> v0/1
  DEC/2(T) -> T/1
  DEC/3(s0) -> s0/1
  DEC/4(a) -> a/1
  DEC/5(b) -> b/1

== system snn_champions_lib/Donatello_LUT64 ==
  s : Inport
  v : Inport  Port=2
  dv : Inport  Port=3
  v_l : Inport  Port=4
  DEC : MATLAB Function  TreatAsAtomicUnit=on
  SNN : MATLAB Function  TreatAsAtomicUnit=on
  v0 : Outport
  T : Outport  Port=2
  s0 : Outport  Port=3
  a : Outport  Port=4
  b : Outport  Port=5
  wires:
  s/1 -> SNN/1(s)
  v/1 -> SNN/2(v)
  dv/1 -> SNN/3(dv)
  v_l/1 -> SNN/4(v_l)
  SNN/1(raw) -> DEC/1(raw)
  SNN/2(valid) -> DEC/2(valid)
  DEC/1(v0) -> v0/1
  DEC/2(T) -> T/1
  DEC/3(s0) -> s0/1
  DEC/4(a) -> a/1
  DEC/5(b) -> b/1

== system snn_champions_lib/Donatello_SLOW ==
  s : Inport
  v : Inport  Port=2
  dv : Inport  Port=3
  v_l : Inport  Port=4
  DEC : MATLAB Function  TreatAsAtomicUnit=on
  SNN : MATLAB Function  TreatAsAtomicUnit=on
  v0 : Outport
  T : Outport  Port=2
  s0 : Outport  Port=3
  a : Outport  Port=4
  b : Outport  Port=5
  wires:
  s/1 -> SNN/1(s)
  v/1 -> SNN/2(v)
  dv/1 -> SNN/3(dv)
  v_l/1 -> SNN/4(v_l)
  SNN/1(raw) -> DEC/1(raw)
  SNN/2(valid) -> DEC/2(valid)
  DEC/1(v0) -> v0/1
  DEC/2(T) -> T/1
  DEC/3(s0) -> s0/1
  DEC/4(a) -> a/1
  DEC/5(b) -> b/1

== system snn_champions_lib/Donatello_Tier ==
  s : Inport
  v : Inport  Port=2
  dv : Inport  Port=3
  v_l : Inport  Port=4
  VS : Subsystem  Variant=on
  v0 : Outport
  T : Outport  Port=2
  s0 : Outport  Port=3
  a : Outport  Port=4
  b : Outport  Port=5
  wires:
  dv/1 -> VS/3(dv)
  s/1 -> VS/1(s)
  v_l/1 -> VS/4(v_l)
  v/1 -> VS/2(v)
  VS/4(a) -> a/1
  VS/1(v0) -> v0/1
  VS/3(s0) -> s0/1
  VS/2(T) -> T/1
  VS/5(b) -> b/1

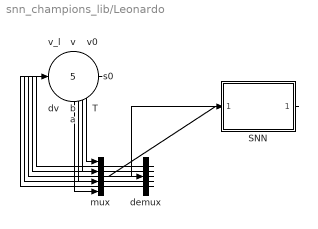
== system snn_champions_lib/Leonardo ==
  s : Inport
  v : Inport  Port=2
  dv : Inport  Port=3
  v_l : Inport  Port=4
  SNN : MATLAB Function  TreatAsAtomicUnit=on
  demux : Demux  Outputs=5
  mux : Mux
  v0 : Outport
  T : Outport  Port=2
  s0 : Outport  Port=3
  a : Outport  Port=4
  b : Outport  Port=5
  wires:
  s/1 -> mux/1
  v/1 -> mux/2
  dv/1 -> mux/3
  v_l/1 -> mux/4
  mux/1 -> SNN/1(x_phys)
  SNN/1(params) -> demux/1
  demux/1 -> v0/1
  demux/2 -> T/1
  demux/3 -> s0/1
  demux/4 -> a/1
  demux/5 -> b/1

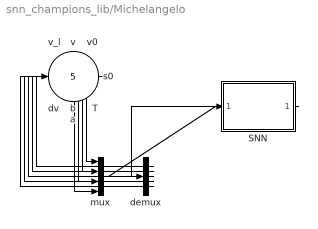
== system snn_champions_lib/Michelangelo ==
  s : Inport
  v : Inport  Port=2
  dv : Inport  Port=3
  v_l : Inport  Port=4
  SNN : MATLAB Function  TreatAsAtomicUnit=on
  demux : Demux  Outputs=5
  mux : Mux
  v0 : Outport
  T : Outport  Port=2
  s0 : Outport  Port=3
  a : Outport  Port=4
  b : Outport  Port=5
  wires:
  s/1 -> mux/1
  v/1 -> mux/2
  dv/1 -> mux/3
  v_l/1 -> mux/4
  mux/1 -> SNN/1(x_phys)
  SNN/1(params) -> demux/1
  demux/1 -> v0/1
  demux/2 -> T/1
  demux/3 -> s0/1
  demux/4 -> a/1
  demux/5 -> b/1

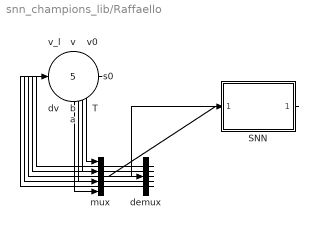
== system snn_champions_lib/Raffaello ==
  s : Inport
  v : Inport  Port=2
  dv : Inport  Port=3
  v_l : Inport  Port=4
  SNN : MATLAB Function  TreatAsAtomicUnit=on
  demux : Demux  Outputs=5
  mux : Mux
  v0 : Outport
  T : Outport  Port=2
  s0 : Outport  Port=3
  a : Outport  Port=4
  b : Outport  Port=5
  wires:
  s/1 -> mux/1
  v/1 -> mux/2
  dv/1 -> mux/3
  v_l/1 -> mux/4
  mux/1 -> SNN/1(x_phys)
  SNN/1(params) -> demux/1
  demux/1 -> v0/1
  demux/2 -> T/1
  demux/3 -> s0/1
  demux/4 -> a/1
  demux/5 -> b/1

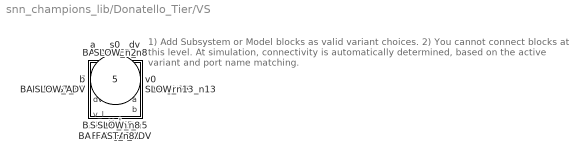
== system snn_champions_lib/Donatello_Tier/VS ==
  note: 1) Add Subsystem or Model blocks as valid variant choices.
      | 2) You cannot connect blocks at this level. At simulation, connectivity is automatically
      | determined, based on the active variant and port name matching.
  s : Inport
  v : Inport  Port=2
  dv : Inport  Port=3
  v_l : Inport  Port=4
  BALANCED_ADV : Subsystem  VariantControl=ADV==1 && TIER==2
  BALANCED_n13 : Subsystem  VariantControl=ADV==0 && TIER==2 && NFRAC==1
  BALANCED_n2 : Subsystem  VariantControl=ADV==0 && TIER==2 && NFRAC==4
  BALANCED_n5 : Subsystem  VariantControl=ADV==0 && TIER==2 && NFRAC==3
  BALANCED_n8 : Subsystem  VariantControl=ADV==0 && TIER==2 && NFRAC==2
  FAST_ADV : Subsystem  VariantControl=ADV==1 && TIER==3
  FAST_n13 : Subsystem  VariantControl=ADV==0 && TIER==3 && NFRAC==1
  FAST_n2 : Subsystem  VariantControl=ADV==0 && TIER==3 && NFRAC==4
  FAST_n5 : Subsystem  VariantControl=ADV==0 && TIER==3 && NFRAC==3
  FAST_n8 : Subsystem  VariantControl=ADV==0 && TIER==3 && NFRAC==2
  SLOW_ADV : Subsystem  VariantControl=ADV==1 && TIER==1
  SLOW_n13 : Subsystem  VariantControl=ADV==0 && TIER==1 && NFRAC==1
  SLOW_n2 : Subsystem  VariantControl=ADV==0 && TIER==1 && NFRAC==4
  SLOW_n5 : Subsystem  VariantControl=ADV==0 && TIER==1 && NFRAC==3
  SLOW_n8 : Subsystem  VariantControl=ADV==0 && TIER==1 && NFRAC==2
  v0 : Outport
  T : Outport  Port=2
  s0 : Outport  Port=3
  a : Outport  Port=4
  b : Outport  Port=5

== system snn_champions_lib/Donatello_Tier/VS/BALANCED_ADV ==
  s : Inport
  v : Inport  Port=2
  dv : Inport  Port=3
  v_l : Inport  Port=4
  DEC : MATLAB Function  TreatAsAtomicUnit=on
  SNN : MATLAB Function  TreatAsAtomicUnit=on
  v0 : Outport
  T : Outport  Port=2
  s0 : Outport  Port=3
  a : Outport  Port=4
  b : Outport  Port=5
  wires:
  s/1 -> SNN/1(s)
  v/1 -> SNN/2(v)
  dv/1 -> SNN/3(dv)
  v_l/1 -> SNN/4(v_l)
  SNN/1(raw) -> DEC/1(raw)
  SNN/2(valid) -> DEC/2(valid)
  DEC/1(v0) -> v0/1
  DEC/2(T) -> T/1
  DEC/3(s0) -> s0/1
  DEC/4(a) -> a/1
  DEC/5(b) -> b/1

== system snn_champions_lib/Donatello_Tier/VS/BALANCED_n13 ==
  s : Inport
  v : Inport  Port=2
  dv : Inport  Port=3
  v_l : Inport  Port=4
  DEC : MATLAB Function  TreatAsAtomicUnit=on
  SNN : MATLAB Function  TreatAsAtomicUnit=on
  v0 : Outport
  T : Outport  Port=2
  s0 : Outport  Port=3
  a : Outport  Port=4
  b : Outport  Port=5
  wires:
  s/1 -> SNN/1(s)
  v/1 -> SNN/2(v)
  dv/1 -> SNN/3(dv)
  v_l/1 -> SNN/4(v_l)
  SNN/1(raw) -> DEC/1(raw)
  SNN/2(valid) -> DEC/2(valid)
  DEC/1(v0) -> v0/1
  DEC/2(T) -> T/1
  DEC/3(s0) -> s0/1
  DEC/4(a) -> a/1
  DEC/5(b) -> b/1

== system snn_champions_lib/Donatello_Tier/VS/BALANCED_n2 ==
  s : Inport
  v : Inport  Port=2
  dv : Inport  Port=3
  v_l : Inport  Port=4
  DEC : MATLAB Function  TreatAsAtomicUnit=on
  SNN : MATLAB Function  TreatAsAtomicUnit=on
  v0 : Outport
  T : Outport  Port=2
  s0 : Outport  Port=3
  a : Outport  Port=4
  b : Outport  Port=5
  wires:
  s/1 -> SNN/1(s)
  v/1 -> SNN/2(v)
  dv/1 -> SNN/3(dv)
  v_l/1 -> SNN/4(v_l)
  SNN/1(raw) -> DEC/1(raw)
  SNN/2(valid) -> DEC/2(valid)
  DEC/1(v0) -> v0/1
  DEC/2(T) -> T/1
  DEC/3(s0) -> s0/1
  DEC/4(a) -> a/1
  DEC/5(b) -> b/1

== system snn_champions_lib/Donatello_Tier/VS/BALANCED_n5 ==
  s : Inport
  v : Inport  Port=2
  dv : Inport  Port=3
  v_l : Inport  Port=4
  DEC : MATLAB Function  TreatAsAtomicUnit=on
  SNN : MATLAB Function  TreatAsAtomicUnit=on
  v0 : Outport
  T : Outport  Port=2
  s0 : Outport  Port=3
  a : Outport  Port=4
  b : Outport  Port=5
  wires:
  s/1 -> SNN/1(s)
  v/1 -> SNN/2(v)
  dv/1 -> SNN/3(dv)
  v_l/1 -> SNN/4(v_l)
  SNN/1(raw) -> DEC/1(raw)
  SNN/2(valid) -> DEC/2(valid)
  DEC/1(v0) -> v0/1
  DEC/2(T) -> T/1
  DEC/3(s0) -> s0/1
  DEC/4(a) -> a/1
  DEC/5(b) -> b/1

== system snn_champions_lib/Donatello_Tier/VS/BALANCED_n8 ==
  s : Inport
  v : Inport  Port=2
  dv : Inport  Port=3
  v_l : Inport  Port=4
  DEC : MATLAB Function  TreatAsAtomicUnit=on
  SNN : MATLAB Function  TreatAsAtomicUnit=on
  v0 : Outport
  T : Outport  Port=2
  s0 : Outport  Port=3
  a : Outport  Port=4
  b : Outport  Port=5
  wires:
  s/1 -> SNN/1(s)
  v/1 -> SNN/2(v)
  dv/1 -> SNN/3(dv)
  v_l/1 -> SNN/4(v_l)
  SNN/1(raw) -> DEC/1(raw)
  SNN/2(valid) -> DEC/2(valid)
  DEC/1(v0) -> v0/1
  DEC/2(T) -> T/1
  DEC/3(s0) -> s0/1
  DEC/4(a) -> a/1
  DEC/5(b) -> b/1

== system snn_champions_lib/Donatello_Tier/VS/FAST_ADV ==
  s : Inport
  v : Inport  Port=2
  dv : Inport  Port=3
  v_l : Inport  Port=4
  DEC : MATLAB Function  TreatAsAtomicUnit=on
  SNN : MATLAB Function  TreatAsAtomicUnit=on
  v0 : Outport
  T : Outport  Port=2
  s0 : Outport  Port=3
  a : Outport  Port=4
  b : Outport  Port=5
  wires:
  s/1 -> SNN/1(s)
  v/1 -> SNN/2(v)
  dv/1 -> SNN/3(dv)
  v_l/1 -> SNN/4(v_l)
  SNN/1(raw) -> DEC/1(raw)
  SNN/2(valid) -> DEC/2(valid)
  DEC/1(v0) -> v0/1
  DEC/2(T) -> T/1
  DEC/3(s0) -> s0/1
  DEC/4(a) -> a/1
  DEC/5(b) -> b/1

== system snn_champions_lib/Donatello_Tier/VS/FAST_n13 ==
  s : Inport
  v : Inport  Port=2
  dv : Inport  Port=3
  v_l : Inport  Port=4
  DEC : MATLAB Function  TreatAsAtomicUnit=on
  SNN : MATLAB Function  TreatAsAtomicUnit=on
  v0 : Outport
  T : Outport  Port=2
  s0 : Outport  Port=3
  a : Outport  Port=4
  b : Outport  Port=5
  wires:
  s/1 -> SNN/1(s)
  v/1 -> SNN/2(v)
  dv/1 -> SNN/3(dv)
  v_l/1 -> SNN/4(v_l)
  SNN/1(raw) -> DEC/1(raw)
  SNN/2(valid) -> DEC/2(valid)
  DEC/1(v0) -> v0/1
  DEC/2(T) -> T/1
  DEC/3(s0) -> s0/1
  DEC/4(a) -> a/1
  DEC/5(b) -> b/1

== system snn_champions_lib/Donatello_Tier/VS/FAST_n2 ==
  s : Inport
  v : Inport  Port=2
  dv : Inport  Port=3
  v_l : Inport  Port=4
  DEC : MATLAB Function  TreatAsAtomicUnit=on
  SNN : MATLAB Function  TreatAsAtomicUnit=on
  v0 : Outport
  T : Outport  Port=2
  s0 : Outport  Port=3
  a : Outport  Port=4
  b : Outport  Port=5
  wires:
  s/1 -> SNN/1(s)
  v/1 -> SNN/2(v)
  dv/1 -> SNN/3(dv)
  v_l/1 -> SNN/4(v_l)
  SNN/1(raw) -> DEC/1(raw)
  SNN/2(valid) -> DEC/2(valid)
  DEC/1(v0) -> v0/1
  DEC/2(T) -> T/1
  DEC/3(s0) -> s0/1
  DEC/4(a) -> a/1
  DEC/5(b) -> b/1
